simulink model "newController"  (R2023a)
settings: Solver=VariableStepAuto  StartTime=0.0  StopTime=10.0  RelTol=1e-3
libraries: ros2lib x65
(part 2 of 2)

== matlab function newController/PID Control2/MATLAB Function ==
  data: pose input; World2Body output
function World2Body= fcn(pose)

poseQuat = [pose(7), pose(4), pose(5), pose(6)];

uPoseQuat = poseQuat./ norm(poseQuat);

World2Body = transpose(quat2rotm(uPoseQuat));

== matlab function newController/Sliding Mode Control1/Subsystem/Calculate Target Velocity/Target Speed calculation ==
  data: posError input; targetSpeed output; curve input
function targetSpeed = fcn(posError, curve)

targetSpeed = zeros(1,6);
if(~length(curve) == 12)
    %params have not yet been assigned / assgined incorrectly
    fprintf("Velo curves not initilized properly! /n");
    return
end

curve = reshape(curve, 2, 6);

%param(1,x) = max control value
%param(2,x) = the error where max control is reached
%velocity curves = param(1,x) * (-cos(error * pi / (2 * param(2,x)))^1/2 + 1)
for i=1:6
    if(posError(i) == 0 || curve(2,i) == 0)
        targetSpeed(i) = 0;
    else
        if(abs(posError(i)) > curve(2,i))
            posError(i) = curve(2,i)*sign(posError(i));
        end
        
        targetSpeed(i) = curve(1, i) * (1-(abs(cos(posError(i)*pi/(2*curve(2,i))))^(1/2)));
       
    end
end

== matlab function newController/Sliding Mode Control1/Subsystem/Error calculator1 ==
  data: currentPos input; targetPos input; error output
function error = fcn(currentPos, targetPos)

error = zeros(1,6);

%World Frame linear error
eWorld = zeros(1,3);

eWorld(1) = currentPos(1) - targetPos(1);
eWorld(2) = currentPos(2) - targetPos(2);
eWorld(3) = currentPos(3) - targetPos(3);

%Quaternion that represents position
currentQuat = [currentPos(7), currentPos(4), currentPos(5), currentPos(6)];

%make it a unit quaternion
unitQuat = currentQuat ./ norm(currentQuat);

%quaternion that we want to be at
setQuat = [targetPos(7), -targetPos(4), -targetPos(5), -targetPos(6)];

uSetQuat = setQuat ./ norm(setQuat);

%multiply the inverse of the unit quat by the set quat to get an error
eQuat = quatmultiply(uSetQuat, conj(unitQuat));
if(eQuat(1) < 0) 
    eQuat = -eQuat;
end

%total rotation angle
w = max(min(eQuat(1),1),-1);
theta = 2 * acos(w);
%sin(theta/2)
s = sqrt(max(1 - w^2,0));
%rotation axis and rotation vector
if s < 1e-6
   eRot = [0 0 0];
else
   axis = eQuat(2:4) / s;
   eRot = theta * axis;
end

theta_mag = norm(eRot);
if theta_mag < 1e-9
   axisError = [0 0 0];
else
   axisError = (sin(theta_mag/2)/theta_mag) * eRot;
end



error(1) = eWorld(1);
error(2) = eWorld(2);
error(3) = eWorld(3);
error(4) = axisError(1);
error(5) = axisError(2);
error(6) = axisError(3);

fprintf("Error:")
disp(error)
end




% error(4) = eVector(1);
% error(5) = eVector(2);
% error(6) = eVector(3);

% function normalizedError = fcn(currentPosition, currentSetPoint)
% 
% normalized = zeros(1,6);
% 
% normalized(1) = -(currentPosition(1) - currentSetPoint(1));
% normalized(2) = -(currentPosition(2) - currentSetPoint(2));
% normalized(3) = -(currentPosition(3) - currentSetPoint(3));
% 
% W2B = [currentPosition(4), currentPosition(5), currentPosition(6), currentPosition(7)];
% setQuat = [currentSetPoint(4), -currentSetPoint(5), -currentSetPoint(6), -currentSetPoint(7)];
% 
% 
% %Talos Heading in Body Frame
% Tbody = [1,0,0,0];
% 
% %Transform from Body 2 World
% B2W = [W2B(1), -W2B(2), -W2B(3), -W2B(4)] / (norm(W2B) ^ 2);
% 
% %Talos Heading in World Frame
% TWorld = quatmultiply(Tbody, B2W);
% 
% %Talos Heading in World Frame Conjugate
% TWorldI = [TWorld(1), -TWorld(2), -TWorld(3), -TWorld(4)];
% 
% %Current Yaw Error
% eQuat = quatmultiply(setQuat, TWorldI);
% 
% % %axis Error
% axisError = [eQuat(2), eQuat(3), eQuat(4)];
% if(eQuat(1) < 0)
%     axisError = -axisError;
% end
% 
% 
% normalized(4) = axisError(1);
% normalized(5) = axisError(2);
% normalized(6) = axisError(3);
% 
% normalizedError = normalized;

== matlab function newController/Sliding Mode Control1/Subsystem/S Block/MATLAB Function ==
  data: PrevSFlipTime input; lambda input; posError input; veloError input; dt input; SFlipTime output; resetMask input; SSign output; prevSSign input
function [SFlipTime, SSign] = fcn(PrevSFlipTime, lambda, posError, veloError, dt, resetMask, prevSSign)


SFlipTime = PrevSFlipTime;
SSign = zeros(6,1);

S = posError + veloError' .* lambda';

for i=1:6
    SSign(i) = sign(S(i));
end


for i=1:6
    if(~resetMask(i))
        if(prevSSign(i) == SSign(i))
            SFlipTime(i) = SFlipTime(i) + SSign(i) * dt;
        else
            SFlipTime(i) = SSign(i) * dt;
        end
    else
        SFlipTime(i) = 0;
    end
end

== matlab function newController/Sliding Mode Control1/Subsystem/SetPointChangedMask ==
  data: targetPos input; setPointChangedMask output; prevTargetPos input
function setPointChangedMask = fcn(targetPos, prevTargetPos)

setPointChangedMask = zeros(6,1);
for i=1:6
    if(targetPos(i) ~= prevTargetPos(i))
        setPointChangedMask(i) = 1;
    else 
        setPointChangedMask(i) = 0;
    end
end

== matlab function newController/Sliding Mode Control1/Subsystem/W2B matrix ==
  data: pose input; World2Body output
function World2Body= fcn(pose)

poseQuat = [pose(7), pose(4), pose(5), pose(6)];

World2Body = transpose(quat2rotm(poseQuat));
